simulink library "delayErrorDetect"  (R2016b)
settings: Solver=VariableStepAuto  StartTime=0.0  StopTime=10.0  RelTol=1e-3
undefined symbols (not defined in the file or in its folder): delayErrorReaction
settings Model: Creator=march  LastModifiedBy=march

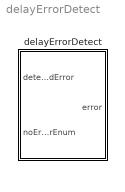
== system delayErrorDetect ==
  delayErrorDetect : Subsystem

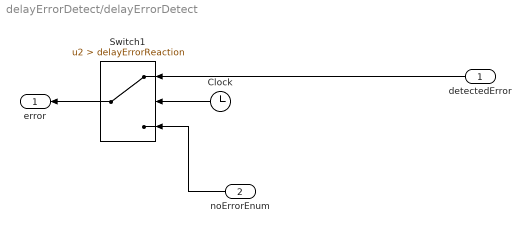
== system delayErrorDetect/delayErrorDetect ==
  detectedError : Inport
  noErrorEnum : Inport  Port=2
  Clock : Clock
  Switch1 : Switch  Criteria=u2 > Threshold  Threshold=delayErrorReaction
  error : Outport
  wires:
  detectedError/1 -> Switch1/1
  noErrorEnum/1 -> Switch1/3
  Clock/1 -> Switch1/2
  Switch1/1 -> error/1
